simulink model "state_regulator"  (R2020a)
settings: Solver=VariableStepAuto  StartTime=0.0  StopTime=30  FixedStep=0.02  RelTol=1e-3  EnableMultiTasking=on
libraries: cstblocks x4
settings Model: ExtModeTrigDuration=10000  Creator=vinja  LastModifiedBy=vinja
settings SolverCC: PositivePriorityOrder=on
settings DataIOCC: ReturnWorkspaceOutputs=off
settings OptimizationCC: LifeSpan=inf
settings DebuggingCC: ArithmeticOperatorsInVariantConditions=warning
settings SFSimCC: SimUseLocalCustomCode=off  CustomCodeUndefinedFunction=UseInterfaceOnly
settings RTWCC: Description=QUARC Win64 Target  SystemTargetFile=quarc_win64.tlc  TemplateMakefile=quarc_default_tmf  RTWUseLocalCustomCode=off
settings CodeAppCC: StateflowObjectComments=on
settings STFCustomTargetCC: TargetPreCompLibLocation=C:\PROGRA~3\QUARC\lib\2020a\win64\release  TargetLangStandard=C99 (ISO)  ConcurrentExecutionCompliant=on  GRTInterface=on  SystemTargetFile=quarc_win64.tlc
settings GRTTargetCC: TargetPreCompLibLocation=C:\PROGRA~3\QUARC\lib\2020a\win64\release  ParMdlRefBuildCompliant=off  CompOptLevelCompliant=off  CombineOutputUpdateFcns=off  MatFileLogging=off  CPPClassGenCompliant=off  GRTInterface=on  UseToolchainInfoCompliant=off  ExtMode=on  ExtModeMexFile=quarc_comm
settings ConfigComp: CovMetricSettings=dswe

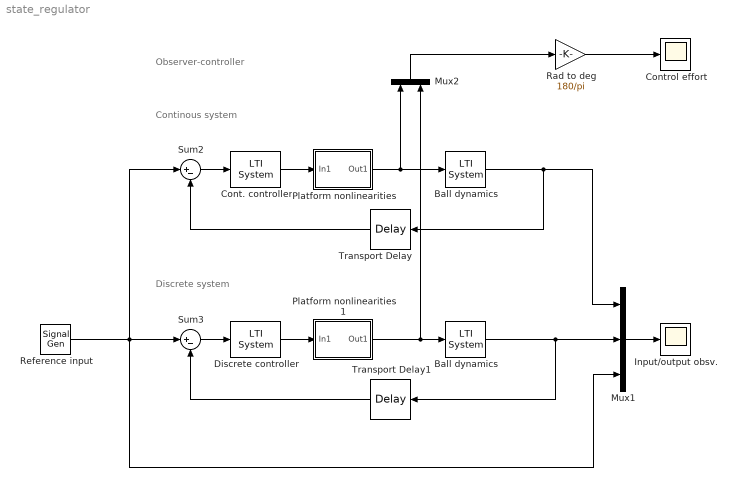
== system state_regulator ==
  note: Observer-controller
  note: Discrete system
  note: Continous system
  Ball dynamics : cstblocks/LTI System  sys=ball  IC=[0.17 0]
  "Ball dynamics " : cstblocks/LTI System  sys=ball  IC=[0.17 0]
  Cont. controller : cstblocks/LTI System  sys=tf_oc  IC=[]
  Control effort : Scope
  Discrete controller : cstblocks/LTI System  sys=tf_oc_d  IC=[]
  Input/output obsv. : Scope
  Mux1 : Mux  Inputs=3
  Mux2 : Mux  Inputs=2
  Platform nonlinearities : Subsystem
  Platform nonlinearities1 : Subsystem
  Rad to deg : Gain  Gain=180/pi
  Reference input : SignalGenerator  WaveForm=square  Amplitude=0  Frequency=0.1
  Sum2 : Sum  Inputs=|+-
  Sum3 : Sum  Inputs=|+-
  Transport Delay : TransportDelay  DelayTime=0.10
  Transport Delay1 : TransportDelay  DelayTime=0.10
  wires:
  Sum2/1 -> Cont. controller/1
  Platform nonlinearities/1(Out1) -> Mux2/1, Ball dynamics/1
  Cont. controller/1 -> Platform nonlinearities/1(In1)
  Rad to deg/1 -> Control effort/1
  "Ball dynamics "/1 -> Mux1/2, Transport Delay1/1
  Discrete controller/1 -> Platform nonlinearities1/1(In1)
  Platform nonlinearities1/1(Out1) -> Mux2/2, "Ball dynamics "/1
  Sum3/1 -> Discrete controller/1
  Mux1/1 -> Input/output obsv./1
  Ball dynamics/1 -> Transport Delay/1, Mux1/1
  Reference input/1 -> Sum2/1, Sum3/1, Mux1/3
  Mux2/1 -> Rad to deg/1
  Transport Delay1/1 -> Sum3/2
  Transport Delay/1 -> Sum2/2

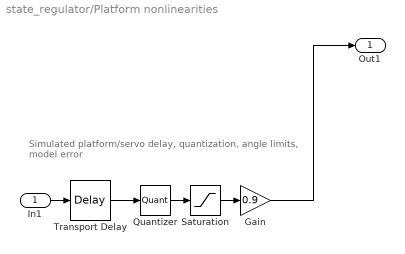
== system state_regulator/Platform nonlinearities ==
  note: Simulated platform/servo delay, quantization, angle limits,
      | model error
  In1 : Inport
  Gain : Gain  Gain=0.9
  Quantizer : Quantizer  QuantizationInterval=pi/256
  Saturation : Saturate  UpperLimit=12.5*pi/180  LowerLimit=-12.5*pi/180
  Transport Delay : TransportDelay  DelayTime=0.08
  Out1 : Outport
  wires:
  Quantizer/1 -> Saturation/1
  Transport Delay/1 -> Quantizer/1
  In1/1 -> Transport Delay/1
  Saturation/1 -> Gain/1
  Gain/1 -> Out1/1

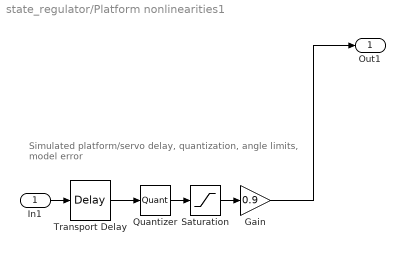
== system state_regulator/Platform nonlinearities1 ==
  note: Simulated platform/servo delay, quantization, angle limits,
      | model error
  In1 : Inport
  Gain : Gain  Gain=0.9
  Quantizer : Quantizer  QuantizationInterval=pi/256
  Saturation : Saturate  UpperLimit=12.5*pi/180  LowerLimit=-12.5*pi/180
  Transport Delay : TransportDelay  DelayTime=0.08
  Out1 : Outport
  wires:
  Quantizer/1 -> Saturation/1
  Transport Delay/1 -> Quantizer/1
  In1/1 -> Transport Delay/1
  Saturation/1 -> Gain/1
  Gain/1 -> Out1/1
